simulink model "generating_data_lane_change"  (R2018b)
settings: Solver=VariableStepAuto  StartTime=0.0  StopTime=Tf  RelTol=1e-3
values from neighbouring files (symbols this model uses):
  T_MPC = 0.1    [main.m]
  throttle_start = 0.02295    [main.m]
  Ts = 0.01    [main.m]
undefined symbols (not defined in the file or in its folder): DiscIntNeverNeededParam, TrackingFunction_lane_change
settings Model: Creator=pm6kgn  LastModifiedBy=t2vosx
settings DebuggingCC: LibraryContextMissingDiagnostic=none
settings SFSimCC: SimUseLocalCustomCode=off
settings RTWCC: RTWUseLocalCustomCode=off

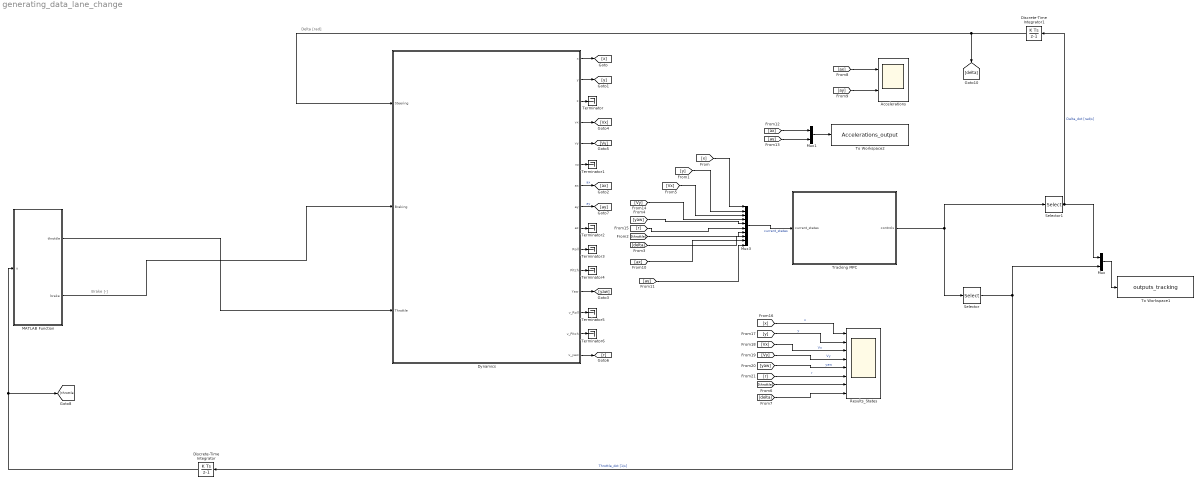
== system generating_data_lane_change ==
  note: Delta [rad]
  note: Brake [-]
  Accelerations : Scope  NumInputPorts=2
  Discrete-Time Integrator : DiscreteIntegrator  InitialCondition=throttle_start  SampleTime=Ts  ICPrevOutput=DiscIntNeverNeededParam  ICPrevScaledInput=DiscIntNeverNeededParam
  Discrete-Time Integrator1 : DiscreteIntegrator  SampleTime=Ts  ICPrevOutput=DiscIntNeverNeededParam  ICPrevScaledInput=DiscIntNeverNeededParam
  Dynamics : Subsystem  Tag=AME2SLCoSim  InitFcn=AMESimLib_initBlock  StartFcn=AMESimLib_startBlock  StopFcn=AMESimLib_stopBlock
      settings: DeleteFcn=AMESimLib_deleteBlock  OpenFcn=AMESimLib_openBlock('AME2SLCoSim')
      mask Display: image(imread('amesim_pix256.png'),[0.4,0.7,0.2,0.2]);disp('Simcenter Amesim co-Sim:\nDynamics');port_label('input',1,'Steering');port_label('input',2,'Braking');port_label('input',3,'Throttle');port_label('output',1,'x');port_label('output',2,'y');port_label('output',3,'z');port_label('output',4,'vx');port_label('output',5,'vy');port_label('output',6,'vz');port_label('output',7,'ax');port_label('output',8,'ay');port_label('output',9,'az');port_label('output',10,'Roll');port_label('output',11,'Pitch');port_label('output',12,'Yaw');port_label('output',13,'v_Roll');port_label('output',14,'v_Pitch');port_label('output',15,'v_yaw');
  MATLAB Function : MATLAB Function  TreatAsAtomicUnit=on  SystemSampleTime=Ts
  Mux : Mux  Inputs=2
  Mux1 : Mux  Inputs=2
  Mux3 : Mux  Inputs=10
  Results_States : Scope  NumInputPorts=8
  Selector : Selector  NumberOfDimensions=2  InputPortWidth=[4 50]  IndexOptions=Index vector (dialog),Index vector (dialog)  Indices=1,1  OutputSizes=1,1
  Selector1 : Selector  NumberOfDimensions=2  InputPortWidth=[4 50]  IndexOptions=Index vector (dialog),Index vector (dialog)  Indices=2,1  OutputSizes=1,1
  Terminator{,1..6} (7 alike) : Terminator
  To Workspace1 : ToWorkspace  VariableName=outputs_tracking  SaveFormat=Structure With Time  SampleTime=-1
  To Workspace2 : ToWorkspace  VariableName=Accelerations_output  SaveFormat=Structure With Time  SampleTime=-1
  Tracking MPC : Subsystem  TreatAsAtomicUnit=on  SystemSampleTime=T_MPC
      mask Display: image('C:\Users\pm6kgn\Documents\Images\2479573.png');
  wires:
  Dynamics/1(x) -> [x]
  Dynamics/4(vx) -> [Vx]
  Dynamics/2(y) -> [y]
  Dynamics/12(Yaw) -> [yaw]
  Dynamics/7(ax) -> [ax]  "ax"
  Dynamics/8(ay) -> [ay]  "ay"
  Selector1/1 -> Discrete-Time Integrator1/1, Mux/1  "Delta_dot [rad/s]"
  Dynamics/5(vy) -> [Vy]
  Dynamics/15(v_yaw) -> [r]
  [x] -> Results_States/1  "x"
  [y] -> Results_States/2  "y"
  [Vx] -> Results_States/3  "Vx"
  [Vy] -> Results_States/4  "Vy"
  [r] -> Results_States/6  "r"
  [yaw] -> Results_States/5  "yaw"
  Tracking MPC/1(controls) -> Selector1/1, Selector/1
  [y] -> Mux3/2
  [x] -> Mux3/1
  Mux3/1 -> Tracking MPC/1("current_states ")  "current_states"
  [Vx] -> Mux3/3
  Dynamics/3(z) -> Terminator/1
  Dynamics/6(vz) -> Terminator1/1
  Dynamics/9(az) -> Terminator2/1
  Dynamics/10(Roll) -> Terminator3/1
  Dynamics/11(Pitch) -> Terminator4/1
  Dynamics/13(v_Roll) -> Terminator5/1
  Dynamics/14(v_Pitch) -> Terminator6/1
  [yaw] -> Mux3/5
  [Vy] -> Mux3/4
  [r] -> Mux3/6
  Selector/1 -> Discrete-Time Integrator/1, Mux/2  "Throttle_dot [1/s]"
  Mux/1 -> To Workspace1/1
  MATLAB Function/1(throttle) -> Dynamics/3(Throttle)
  MATLAB Function/2(brake) -> Dynamics/2(Braking)
  Discrete-Time Integrator1/1 -> [delta], Dynamics/1(Steering)
  [throttle] -> Mux3/7
  [delta] -> Mux3/8
  [ax] -> Accelerations/1
  [ay] -> Accelerations/2
  Discrete-Time Integrator/1 -> MATLAB Function/1(u), [throttle]
  [throttle] -> Results_States/7
  [delta] -> Results_States/8
  [ax] -> Mux3/9
  [ay] -> Mux3/10
  Mux1/1 -> To Workspace2/1
  [ax] -> Mux1/1
  [ay] -> Mux1/2

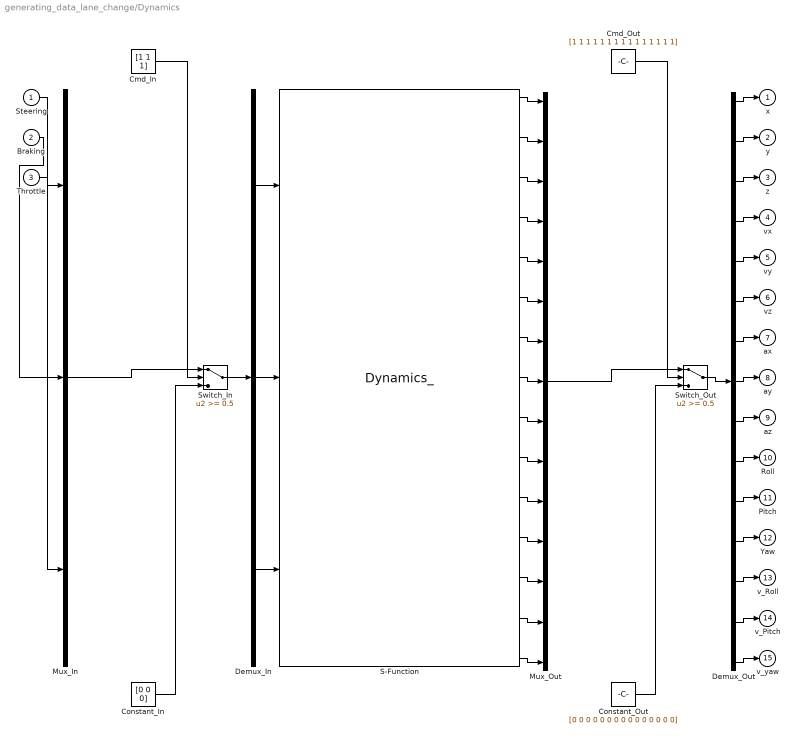
== system generating_data_lane_change/Dynamics ==
  Steering : Inport
  Braking : Inport  Port=2
  Throttle : Inport  Port=3
  Cmd_In : Constant  Value=[1 1 1]
  Cmd_Out : Constant  Value=[1 1 1 1 1 1 1 1 1 1 1 1 1 1 1]
  Constant_In : Constant  Value=[0 0 0]
  Constant_Out : Constant  Value=[0 0 0 0 0 0 0 0 0 0 0 0 0 0 0]
  Demux_In : Demux  Outputs=3
  Demux_Out : Demux  Outputs=15
  Mux_In : Mux  Inputs=3
  Mux_Out : Mux  Inputs=15
  S-Function : S-Function  InitFcn=clear Dynamics_  StopFcn=clear Dynamics_  FunctionName=Dynamics_  Parameters="[0.01;0.01;1e-05;1e+30;100;0;0;2;0;1;0.001;0;1] ['Grav           ';'Xg             ';'Zg             ';'V0             ';'Msprung        ';'Msteer         ';'Msp_front      ';'Mwh_front      ';'Msp_rear       ';'Mwh_rear       ';'Isprung_xx     ';'Isprung_yy     ';'Isprung_zz     ';'Isprung_xy     ';'Isprung_xz     ';'Isprung_yz     ';'Zref_front     ';'Zref_rear      ';'wheelbase      ';'track_front    ';'track_rear     ';'Rpinion        ';'Ksusp_front    ';'Ksusp_rear     ';'Rsusp_front    ';'Rsusp_rear     ';'Kantiroll_front';'Kantiroll_rear ';'Rfree          ';'Rroll          ';'Ktire          ';'Rtire          ';'a1             ';'a2             ';'a3             ';'a4             '] [9.8066;1056;375;22.2222;1300;2;18;18;15;14;250;1000;1300;0;-20;0;75;75;2400;1450;1450;8;21000;21000;2000;1500;30000;20000;0.292;0.291;200000;100;-50;1200;1000;5] [] [] [] []"  SFunctionDeploymentMode=off  EnableBusSupport=off
      mask Display: port_label('output',1,'x');port_label('output',2,'y');port_label('output',3,'z');port_label('output',4,'vx');port_label('output',5,'vy');port_label('output',6,'vz');port_label('output',7,'ax');port_label('output',8,'ay');port_label('output',9,'az');port_label('output',10,'Roll');port_label('output',11,'Pitch');port_label('output',12,'Yaw');port_label('output',13,'v_Roll');port_label('output',14,'v_Pitch');port_label('output',15,'v_yaw');port_label('input',1,'Steering');port_label('input',2,'Braking');port_label('input',3,'Throttle');disp('Simcenter Amesim:\n Dynamics_')
  Switch_In : Switch  Threshold=0.5  SaturateOnIntegerOverflow=on  InputSameDT=on
  Switch_Out : Switch  Threshold=0.5  SaturateOnIntegerOverflow=on  InputSameDT=on
  x : Outport
  y : Outport  Port=2
  z : Outport  Port=3
  vx : Outport  Port=4
  vy : Outport  Port=5
  vz : Outport  Port=6
  ax : Outport  Port=7
  ay : Outport  Port=8
  az : Outport  Port=9
  Roll : Outport  Port=10
  Pitch : Outport  Port=11
  Yaw : Outport  Port=12
  v_Roll : Outport  Port=13
  v_Pitch : Outport  Port=14
  v_yaw : Outport  Port=15
  wires:
  Mux_In/1 -> Switch_In/1
  Cmd_In/1 -> Switch_In/2
  Constant_In/1 -> Switch_In/3
  Switch_In/1 -> Demux_In/1
  Mux_Out/1 -> Switch_Out/1
  Cmd_Out/1 -> Switch_Out/2
  Constant_Out/1 -> Switch_Out/3
  Switch_Out/1 -> Demux_Out/1
  Steering/1 -> Mux_In/1
  Demux_In/1 -> S-Function/1
  Braking/1 -> Mux_In/2
  Demux_In/2 -> S-Function/2
  Throttle/1 -> Mux_In/3
  Demux_In/3 -> S-Function/3
  Demux_Out/1 -> x/1
  S-Function/1 -> Mux_Out/1
  Demux_Out/2 -> y/1
  S-Function/2 -> Mux_Out/2
  Demux_Out/3 -> z/1
  S-Function/3 -> Mux_Out/3
  Demux_Out/4 -> vx/1
  S-Function/4 -> Mux_Out/4
  Demux_Out/5 -> vy/1
  S-Function/5 -> Mux_Out/5
  Demux_Out/6 -> vz/1
  S-Function/6 -> Mux_Out/6
  Demux_Out/7 -> ax/1
  S-Function/7 -> Mux_Out/7
  Demux_Out/8 -> ay/1
  S-Function/8 -> Mux_Out/8
  Demux_Out/9 -> az/1
  S-Function/9 -> Mux_Out/9
  Demux_Out/10 -> Roll/1
  S-Function/10 -> Mux_Out/10
  Demux_Out/11 -> Pitch/1
  S-Function/11 -> Mux_Out/11
  Demux_Out/12 -> Yaw/1
  S-Function/12 -> Mux_Out/12
  Demux_Out/13 -> v_Roll/1
  S-Function/13 -> Mux_Out/13
  Demux_Out/14 -> v_Pitch/1
  S-Function/14 -> Mux_Out/14
  Demux_Out/15 -> v_yaw/1
  S-Function/15 -> Mux_Out/15

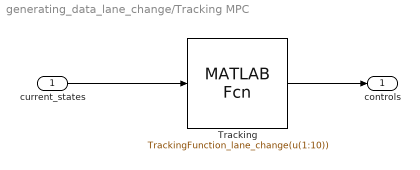
== system generating_data_lane_change/Tracking MPC ==
  "current_states " : Inport
  Tracking : MATLABFcn  MATLABFcn=TrackingFunction_lane_change(u(1:10))  OutputDimensions=[2,1]  Output1D=off
  controls : Outport
  wires:
  Tracking/1 -> controls/1
  "current_states "/1 -> Tracking/1

== matlab function generating_data_lane_change/MATLAB Function ==
  data: u input; throttle output; brake output
function [throttle, brake]= fcn(u)

    if u >= 0
        throttle = u;
        brake = 0;
    else
        brake = u;
        throttle = 0;
    end

end
